simulink model "mlf_distpipe"  (R2015b)
settings: Solver=FixedStepDiscrete  SolverMode=SingleTasking  StartTime=0.0  StopTime=10  RelTol=1e-3
libraries: simulink x3
settings Model: Creator=at-mt  LastModifiedBy=amatsumo
settings DataIOCC: SaveFormat=Array  SignalLoggingSaveFormat=ModelDataLogs  SaveOutput=off  SignalLogging=off  SaveTime=off
settings OptimizationCC: BlockReduction=off  ConditionallyExecuteInputs=off  DefaultParameterBehavior=Inlined  ExpressionDepthLimit=2147483647
settings DebuggingCC: AlgebraicLoopMsg=error  UnderspecifiedInitializationDetection=Classic  MergeDetectMultiDrivingBlocksExec=none  SolverPrmCheckMsg=warning  SingleTaskRateTransMsg=error  FcnCallInpInsideContextMsg=UseLocalSettings  StateNameClashWarn=warning
settings HardwareCC: ProdBitPerPointer=32  ProdLargestAtomicFloat=None  ProdIntDivRoundTo=Undefined  ProdEndianess=Unspecified  ProdWordSize=32  ProdHWDeviceType=ASIC/FPGA->ASIC/FPGA  ProdEqTarget=off
settings SFSimCC: SFSimEcho=off
settings RTWCC: GenerateReport=on  LaunchReport=on
settings GRTTargetCC: GeneratePreprocessorConditionals=Disable all  CombineOutputUpdateFcns=off  GRTInterface=on
settings ConfigComp: CovModelRefEnable=Off  CovSFcnEnable=off

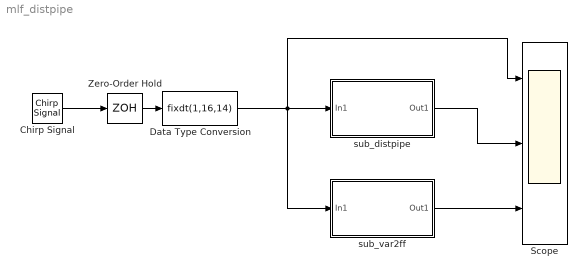
== system mlf_distpipe ==
  Chirp Signal : simulink/Sources/Chirp Signal  f1=10  T=10  f2=500
  Data Type Conversion : DataTypeConversion  OutDataTypeStr=fixdt(1,16,14)
  Scope : Scope  NumInputPorts=3
  Zero-Order Hold : ZeroOrderHold  SampleTime=1/1000
  sub_distpipe : Subsystem
  sub_var2ff : Subsystem
  wires:
  Chirp Signal/1 -> Zero-Order Hold/1
  Zero-Order Hold/1 -> Data Type Conversion/1
  Data Type Conversion/1 -> sub_var2ff/1(In1), Scope/1, sub_distpipe/1(In1)
  sub_distpipe/1(Out1) -> Scope/2
  sub_var2ff/1(Out1) -> Scope/3

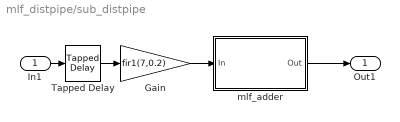
== system mlf_distpipe/sub_distpipe ==
  In1 : Inport
  Gain : Gain  Gain=fir1(7,0.2)  ParamDataTypeStr=fixdt(1,16,16)  OutDataTypeStr=Inherit: Same as input
  Tapped Delay : simulink/Discrete/Tapped Delay  vinit=0.0  samptime=-1  NumDelays=7  DelayOrder=Newest  includeCurrent=on
  mlf_adder : MATLAB Function  TreatAsAtomicUnit=on
  Out1 : Outport
  wires:
  mlf_adder/1(Out) -> Out1/1
  In1/1 -> Tapped Delay/1
  Tapped Delay/1 -> Gain/1
  Gain/1 -> mlf_adder/1(In)

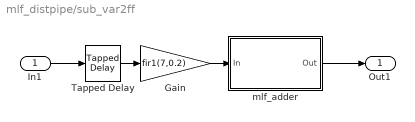
== system mlf_distpipe/sub_var2ff ==
  In1 : Inport
  Gain : Gain  Gain=fir1(7,0.2)  ParamDataTypeStr=fixdt(1,16,16)  OutDataTypeStr=Inherit: Same as input
  Tapped Delay : simulink/Discrete/Tapped Delay  vinit=0.0  samptime=-1  NumDelays=7  DelayOrder=Newest  includeCurrent=on
  mlf_adder : MATLAB Function  TreatAsAtomicUnit=on
  Out1 : Outport
  wires:
  Tapped Delay/1 -> Gain/1
  In1/1 -> Tapped Delay/1
  mlf_adder/1(Out) -> Out1/1
  Gain/1 -> mlf_adder/1(In)

== matlab function mlf_distpipe/sub_distpipe/mlf_adder ==
  settings: fimath=|
      | fimath(...
      | 'RoundMode', 'floor',...
      | 'OverflowMode', 'wrap',...
      | 'ProductMode', 'KeepLSB', 'ProductWordLength', 32,...
      | 'SumMode', 'KeepLSB', 'SumWordLength', 32,...
      | 'CastBeforeSum', true)
      | 
      | %hdlfimath;
  data: In input; Out output
function Out = fcn(In)


% stage 0 to 1
y1 = In(1)+In(2);
y2 = In(3)+In(4);
y3 = In(5)+In(6);
y4 = In(7)+In(8);

% stage 1 to 2
y5 = y1+y2;
y6 = y3+y4;

% stage 2 to 3
Out =fi(y5+y6, 1,16,14);

== matlab function mlf_distpipe/sub_var2ff/mlf_adder ==
  settings: fimath=hdlfimath;
  data: In input; Out output
function Out = fcn(In)

buf1 = fi(zeros(1,4), 1, 17, 14);	% pre allocation
buf2 = fi(zeros(1,2), 1, 18, 14);  % pre allocation

% stage 0 to 1
buf1(1) = In(1)+In(2);
buf1(2) = In(3)+In(4);
buf1(3) = In(5)+In(6);
buf1(4) = In(7)+In(8);

% stage 1 to 2
buf2(1) = buf1(1)+buf1(2);
buf2(2) = buf1(3)+buf1(4);

% stage 2 to 3
Out =fi(sum(buf2), 1,16,14);
